simulink model "My_ESP_Model"  (R2021a)
settings: Solver=VariableStepAuto  StartTime=0.0  StopTime=30.0  MaxStep=1e-3  RelTol=1e-3
values from neighbouring files (symbols this model uses):
  H = [ones(1,4) ... (first row only)    [NL_Main.m]
  lambda0 = [lambda0s; lambda0s; 0; 0]    [NL_Main.m]
  u0 = [lambda0; delta_r0]    [NL_Main.m]
  v0x = v0*cos(beta0)    [NL_Main.m]
  x0 = 0    [NL_Main.m]
undefined symbols (not defined in the file or in its folder): B1_lambda, delta_f, kest, Kr, pinv
settings Model: Creator=patta  LastModifiedBy=miche
settings SolverCC: AlgebraicLoopSolver=TrustRegion
settings DataIOCC: ReturnWorkspaceOutputs=off
settings DebuggingCC: SFMachineParentedDataDiag=warning  UnderSpecifiedDimensionMsg=warning  ArithmeticOperatorsInVariantConditions=warning
settings SFSimCC: CustomCodeUndefinedFunction=UseInterfaceOnly

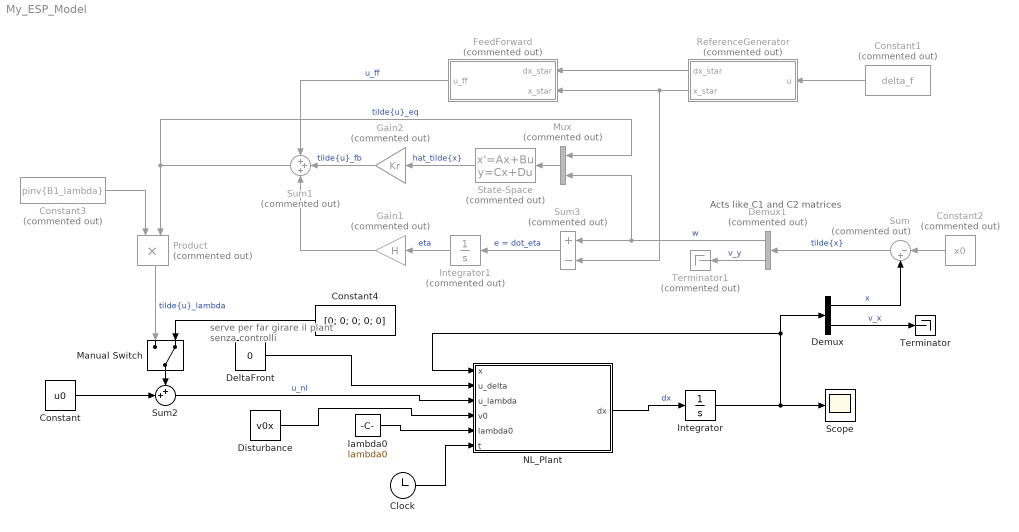
== system My_ESP_Model ==
  note: serve per far girare il plant senza controlli
  note: Acts like C1 and C2 matrices
  Clock : Clock
  Constant : Constant  Value=u0  VectorParams1D=off
  Constant1 : Constant  Commented=on  Value=delta_f
  Constant2 : Constant  Commented=on  Value=x0
  Constant3 : Constant  Commented=on  Value=pinv{B1_lambda}
  Constant4 : Constant  Value=[0; 0; 0; 0; 0]
  DeltaFront : Constant  Value=0
  Demux : Demux  Outputs=2
  Demux1 : Demux  Commented=on  Outputs=2
  Disturbance : Constant  Value=v0x
  FeedForward : MATLAB Function  Commented=on  TreatAsAtomicUnit=on
  Gain1 : Gain  Commented=on  Gain=H
  Gain2 : Gain  Commented=on  Gain=Kr
  Integrator : Integrator  InitialCondition=[5; 0; 0]
  Integrator1 : Integrator  Commented=on
  Manual Switch : ManualSwitch  CurrentSetting=0
  Mux : Mux  Commented=on  Inputs=2
  NL_Plant : MATLAB Function  TreatAsAtomicUnit=on
  Product : Product  Commented=on
  ReferenceGenerator : MATLAB Function  Commented=on  TreatAsAtomicUnit=on
  Scope : Scope
  State-Space : StateSpace  Commented=on  A=kest.A  B=kest.B  C=kest.C(2:end,:)  D=kest.D(2:end,:)  InitialCondition=0
  Sum : Sum  Commented=on  Inputs=|-+
  Sum1 : Sum  Commented=on  Inputs=+++
  Sum2 : Sum  Inputs=++|
  Sum3 : Sum  Commented=on  Inputs=+-
  Terminator : Terminator
  Terminator1 : Terminator  Commented=on
  lambda0 : Constant  Value=lambda0
  wires:
  NL_Plant/1(dx) -> Integrator/1  "dx"
  Integrator/1 -> Demux/1, NL_Plant/1(x), Scope/1
  Disturbance/1 -> NL_Plant/4(v0)
  State-Space/1 -> Gain2/1  "hat_tilde{x}"
  Gain2/1 -> Sum1/2  "tilde{u}_fb"
  Sum/1 -> Demux1/1  "tilde{x}"
  Integrator1/1 -> Gain1/1  "eta"
  ReferenceGenerator/2(x_star) -> FeedForward/2(x_star), Sum3/2
  Constant1/1 -> ReferenceGenerator/1(u)
  Sum1/1 -> Product/2, Mux/1  "tilde{u}_eq"
  Gain1/1 -> Sum1/3
  FeedForward/1(u_ff) -> Sum1/1  "u_ff"
  ReferenceGenerator/1(dx_star) -> FeedForward/1(dx_star)
  lambda0/1 -> NL_Plant/5(lambda0)
  Demux/1 -> Sum/2  "x"
  Sum3/1 -> Integrator1/1  "e = dot_eta"
  Mux/1 -> State-Space/1
  Demux/2 -> Terminator/1  "v_x"
  Constant2/1 -> Sum/1
  Constant3/1 -> Product/1
  Demux1/2 -> Terminator1/1  "v_y"
  Demux1/1 -> Sum3/1, Mux/2  "w"
  Sum2/1 -> NL_Plant/3(u_lambda)  "u_nl"
  Constant/1 -> Sum2/2
  Product/1 -> Manual Switch/1  "tilde{u}_lambda"
  Manual Switch/1 -> Sum2/1
  Constant4/1 -> Manual Switch/2
  DeltaFront/1 -> NL_Plant/2(u_delta)
  Clock/1 -> NL_Plant/6(t)

== matlab function My_ESP_Model/ReferenceGenerator ==
  data: dx_star output; u input; x_star output
function [dx_star,x_star] = RefGen(u)
g = 9.81; % [m/s^2] gravity acceleration
rho = 1.225; % [kg/m^3] air density
S = 2.4; % [m^2] cross surface
Cx0 = -0.3; % [-] drag coefficient
Cyb = -0.3; % [-] drag coefficient
rk = 1; % dry asphalt
m = 1200; % [kg] vehicle mass
rxf = 1.4;
rxr = -0.5;
ryf = 0.90;
rz =  0.70;
CR = -0.05;
Iz = 1200*(rxr^2 + ryf^2)^2;

delta = 0*[1 1 0 0]/180*pi; % 3.5 // 10

rx = [rxf rxf rxr rxr];
ry = [ryf -ryf -ryf ryf];
H = [ones(1,4);
    ry;
    -rx];

%% EQUILIBRIUM POINT
%  global v0 FzW
x0 = 0;
y0 = 0;
v0 = 270/3.6; % [m/s] vehicle speed
beta0 = 0;
w0 = 0;
psi0 = 0/180*pi;
theta = 15/180*pi;

end

%% Mu

function mu = mu_long(i,lambda)

% 1) Dry asphalt
% 2) wet asphalt
% 3) Snow
% 4) Ice
% 5) Dry Cobblestone
% 6) wet cobblestone
theta1 = [1.28 0.86 0.19 0.05 1.37 0.4];
theta2 = [23.99 33.82 94.13 306.39 6.46 33.71];
theta3 = [0.52 0.35 0.05 0 0.67 0.12];

mu = sign(lambda).*theta1(i).*(1-exp(-abs(lambda)*theta2(i)))-theta3(i)*lambda;

end

% Partial derivative of mu
function mu = Partial_mu_long(i,lambda)

% 1) Dry asphalt
% 2) wet asphalt
% 3) Snow
% 4) Ice
% 5) Dry Cobblestone
% 6) wet cobblestone
theta1 = [1.28 0.86 0.19 0.05 1.37 0.4];
theta2 = [23.99 33.82 94.13 306.39 6.46 33.71];
theta3 = [0.52 0.35 0.05 0 0.67 0.12];

mu = theta1(i).*theta2(i).*exp(-abs(lambda).*theta2(i))-theta3(i);

end

== matlab function My_ESP_Model/NL_Plant ==
  data: x input; dx output; u_delta input; u_lambda input; v0 input; lambda0 input; t input
function dx = NLPlant(x,u_delta,u_lambda,v0,lambda0,t)

%  HAS THE LAMBDAS STILL TO BE CONSIDERED AT "0" VALUE VALUE??

g = 9.81; % [m/s^2] gravity acceleration
rho = 1.225; % [kg/m^3] air density
S = 2.4; % [m^2] cross surface
Cd = -0.3; % [-] drag coefficient
rk = 1; % dry asphalt
m = 1200; % [kg] vehicle mass
rxf = 1.4;
rxr = -0.5;
ryf = 0.90;
rz =  0.70;
CR = -0.05;
Iz = 1200*(rxr^2 + ryf^2)^2;
beta = pi/16; % Inserito manualmente

delta0 = 0*[1 1 0 0]/180*pi; % 3.5 // 10

w = x(1);
v_y = x(2);

rx = [rxf rxf rxr rxr];
ry = [ryf -ryf -ryf ryf];
H = [ones(1,4);
    -rx;
     ry];

%% NON LINEAR EQUATIONS

v = v0;
v_y = v*sin(beta);

delta = SteeringWheel(t).*[1 1 0 0]; % Per definire la matrice dei delta, altrimenti viene un elemento solo
% deltaW iesimo è definito tramite una catena cinematica calcolata nella
% funzione SteeringWheel; credo che bisogni definirla poi un altra per le
% route posteriori?
pinvH = pinv(H);

tau = 0;
fB_x = 0;
fB_y = 0;
FzW = pinvH*[m*g; rz/2*rho*S*v^2; 0]; % Cm*l is also needed
ryi = 0;
rxi = 0;
vWi = 0;
vW_xi = 0;
vW_yi = 0;
betai = 0;
mu_lambdai = 0;
mu_betai = 0;
fW_xi = 0;
fW_yi =0;
% let's start to build the equations from the 12.1f
for i = 1:4 % looping for each tyre 
   
    deltai = delta(i);
    
    ryi = ry(i);
    rxi = rx(i);
    % speed in the reference system of the wheel to compute
    % the side slip angle beta
    vWi = [cos(deltai) sin(deltai);
        -sin(deltai) cos(deltai)]*(w*[-ryi; rxi]+[v_y; v*cos(beta)]);
    vW_xi = vWi(1);
    vW_yi = vWi(2);
    betai = -atan(vW_yi/vW_xi);
    % settings for the type of asphalt in the mu equation   
    
    mu_lambdai = mu_long(rk,lambda0(i)); %mu with lambdas (longitudinal slip angle)
    mu_betai = -mu_long(rk,betai); % mu with betas (side slip angle)
    
    fW_xi = mu_lambdai*FzW(i);
    fW_yi = mu_betai*FzW(i);
    
    fB_x = fB_x + [cos(deltai) -sin(deltai)]*[fW_xi; fW_yi];
    fB_y = fB_y + [sin(deltai) cos(deltai)]*[fW_xi; fW_yi];
    tau = tau + ([sin(deltai) -cos(deltai)].*ryi)*[fW_yi; fW_xi] + ([sin(deltai) cos(deltai)].*rxi)*[fW_xi; fW_yi];
end

dx =[m^(-1)*(fB_x + m*w*v*sin(beta) - 1/2*rho*S*v^2*Cd);
     m^(-1)*(fB_y - m*w*v*cos(beta));
     Iz^(-1)*tau];

end


%% used functions
function mu = mu_long(i,lambda)

% 1) Dry asphalt
% 2) wet asphalt
% 3) Snow
% 4) Ice
% 5) Dry Cobblestone
% 6) wet cobblestone
theta1 = [1.28 0.86 0.19 0.05 1.37 0.4];
theta2 = [23.99 33.82 94.13 306.39 6.46 33.71];
theta3 = [0.52 0.35 0.05 0 0.67 0.12];

mu = sign(lambda).*theta1(i).*(1-exp(-abs(lambda)*theta2(i)))-theta3(i)*lambda;

end

% Partial derivative of mu
function mu = Partial_mu_long(i,lambda)

% 1) Dry asphalt
% 2) wet asphalt
% 3) Snow
% 4) Ice
% 5) Dry Cobblestone
% 6) wet cobblestone
theta1 = [1.28 0.86 0.19 0.05 1.37 0.4];
theta2 = [23.99 33.82 94.13 306.39 6.46 33.71];
theta3 = [0.52 0.35 0.05 0 0.67 0.12];

mu = theta1(i).*theta2(i).*exp(-abs(lambda).*theta2(i))-theta3(i);

end

function delta_f = SteeringWheel(t)

ti = 5; % [s] inital time
tf = 7; % [s] final time
A = 5/180*pi; %[rad] steering wheel maximum amplitude
%FaB = 1/2*rho*S*v^2*Cd;

type = 0;
% 0 = sin
% 1 = step

switch type
    case 0
        % SIN COMPUTATION
        DT = tf-ti; % [s] steering action duration
        w = 2*pi/DT;
        
        if t >= ti && t <= tf
            delta_f = A*sin(w*(t-ti));
        else
            delta_f = 0;
        end
    case 1
        if t >= ti 
            delta_f = A;
        else
            delta_f = 0;
        end
end
end

== matlab function My_ESP_Model/FeedForward ==
  data: dx_star input; x_star input; u_ff output
function u_ff = FFNet (dx_star, x_star)

g = 9.81; % [m/s^2] gravity acceleration
rho = 1.225; % [kg/m^3] air density
S = 2.4; % [m^2] cross surface
Cx0 = -0.3; % [-] drag coefficient
Cyb = -0.3; % [-] drag coefficient
rk = 1; % dry asphalt
m = 1200; % [kg] vehicle mass
rxf = 1.4;
rxr = -0.5;
ryf = 0.90;
rz =  0.70;
CR = -0.05;
Iz = 1200*(rxr^2 + ryf^2)^2;

delta = 0*[1 1 0 0]/180*pi; % 3.5 // 10

rx = [rxf rxf rxr rxr];
ry = [ryf -ryf -ryf ryf];
H = [ones(1,4);
    ry;
    -rx];

%% EQUILIBRIUM POINT
%  global v0 FzW
x0 = 0;
y0 = 0;
v0 = 270/3.6; % [m/s] vehicle speed
beta0 = 0;
w0 = 0;
psi0 = 0/180*pi;
theta = 15/180*pi;

end

%% Mu

function mu = mu_long(i,lambda)

% 1) Dry asphalt
% 2) wet asphalt
% 3) Snow
% 4) Ice
% 5) Dry Cobblestone
% 6) wet cobblestone
theta1 = [1.28 0.86 0.19 0.05 1.37 0.4];
theta2 = [23.99 33.82 94.13 306.39 6.46 33.71];
theta3 = [0.52 0.35 0.05 0 0.67 0.12];

mu = sign(lambda).*theta1(i).*(1-exp(-abs(lambda)*theta2(i)))-theta3(i)*lambda;

end

% Partial derivative of mu
function mu = Partial_mu_long(i,lambda)

% 1) Dry asphalt
% 2) wet asphalt
% 3) Snow
% 4) Ice
% 5) Dry Cobblestone
% 6) wet cobblestone
theta1 = [1.28 0.86 0.19 0.05 1.37 0.4];
theta2 = [23.99 33.82 94.13 306.39 6.46 33.71];
theta3 = [0.52 0.35 0.05 0 0.67 0.12];

mu = theta1(i).*theta2(i).*exp(-abs(lambda).*theta2(i))-theta3(i);

end
